simulink model "Environment"  (R2025b)
settings: Solver=FixedStepAuto  StartTime=0.0  StopTime=50  FixedStep=0.01  RelTol=1e-3
libraries: aerolibasang x2, aerolibwind2 x1, aerolibatmos2 x1
settings Model: DataDictionary=Environment_data.sldd  Creator=mauro  LastModifiedBy=mauro

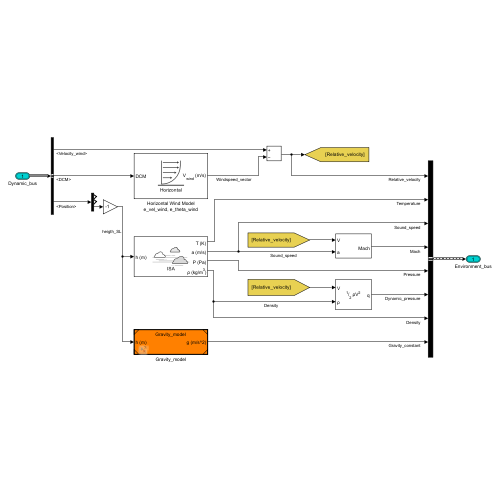
[thumbnail: Simulink's stored preview of the top-level diagram]
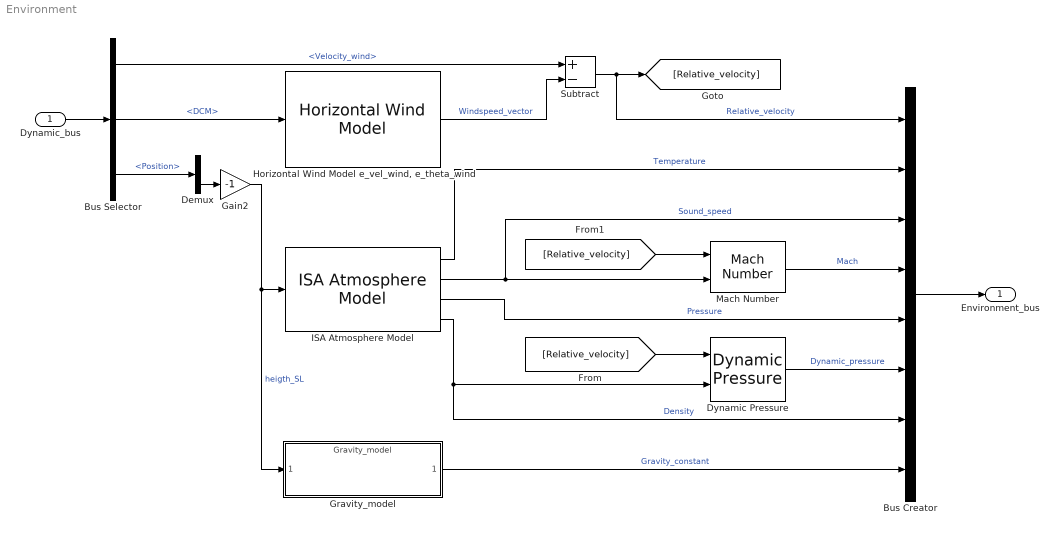
== system Environment ==
  Dynamic_bus : Inport  OutDataTypeStr=Bus: Dynamic_bus
  Bus Creator : BusCreator  Inputs=8  OutDataTypeStr=Bus: Environment_bus  NonVirtualBus=on
  Bus Selector : BusSelector  OutputSignals=Velocity_wind,DCM,Position
  Demux : Demux  Outputs=3
  Dynamic Pressure : aerolibasang/Dynamic Pressure
  Gain2 : Gain  Gain=-1
  Gravity_model : ModelReference  ModelNameDialog=Gravity_model.slx  SimulationMode=Normal  ModelReferenceVersion=1.13
  "Horizontal Wind Model e_vel_wind, e_theta_wind" : aerolibwind2/Horizontal Wind Model  units=Metric (MKS)  Vw_source=Internal  Vwind=e_vel_wind  W_source=Internal  Wdeg=e_theta_wind
  ISA Atmosphere Model : aerolibatmos2/ISA Atmosphere Model  useExtended=off  action=None  custom=off  viscosityOut=off  g=9.80665  gamma=1.4  R=287.0531  L=0.0065  h_trop=11000  h_strat=20000  rho0=1.225  P0=101325  T0=288.15  h0=0  S=110.4  Tref=273.15  muref=1.716e-5
  Mach Number : aerolibasang/Mach Number
  Subtract : Sum  Inputs=+-
  Environment_bus : Outport  OutDataTypeStr=Bus: Environment_bus  BusOutputAsStruct=on
  wires:
  Gain2/1 -> Gravity_model/1, ISA Atmosphere Model/1  "heigth_SL"
  ISA Atmosphere Model/4 -> Dynamic Pressure/2, Bus Creator/7  "Density"
  [Relative_velocity] -> Dynamic Pressure/1
  ISA Atmosphere Model/2 -> Bus Creator/3, Mach Number/2  "Sound_speed"
  "Horizontal Wind Model e_vel_wind, e_theta_wind"/1 -> Subtract/2  "Windspeed_vector"
  ISA Atmosphere Model/1 -> Bus Creator/2  "Temperature"
  Mach Number/1 -> Bus Creator/4  "Mach"
  ISA Atmosphere Model/3 -> Bus Creator/5  "Pressure"
  Dynamic Pressure/1 -> Bus Creator/6  "Dynamic_pressure"
  Gravity_model/1 -> Bus Creator/8  "Gravity_constant"
  Subtract/1 -> Bus Creator/1, [Relative_velocity]  "Relative_velocity"
  [Relative_velocity] -> Mach Number/1
  Bus Creator/1 -> Environment_bus/1
  Dynamic_bus/1 -> Bus Selector/1
  Bus Selector/1 -> Subtract/1  "<Velocity_wind>"
  Bus Selector/2 -> "Horizontal Wind Model e_vel_wind, e_theta_wind"/1  "<DCM>"
  Bus Selector/3 -> Demux/1  "<Position>"
  Demux/3 -> Gain2/1
